simulink model "rlAgentLCLatConstantVxSUMO"  (R2024a)
settings: Solver=VariableStepAuto  StartTime=0.0  StopTime=Tf  FixedStep=1e-3  MaxStep=0.1  RelTol=1e-3
values from neighbouring files (symbols this model uses):
  A = [0 0 0 0 1 -43.6764705882 0 -6.44154540893 0 436.764705882 0 64.4154540893 ... (16 elements, 4x4)]    [DDPGTrain4PingWang.mat]    (also in rlAgentLCParams.m = [)
  Alo = [0  1; 0  0]    [DDPGTrain1.mat]    (also in DDPGTrain2.mat; DDPGTrain4PingWang.mat; rlAgentLCParams.m = [0 1; 0 0])
  B = [0 222.058823529 0 219.719016558]    [DDPGTrain4PingWang.mat]    (also in rlAgentLCParams.m = [0 2*Cf/m 0 2*lf*Cf/Iz]')
  Blo = [0 0.000735294117647]    [DDPGTrain1.mat]    (also in DDPGTrain2.mat; DDPGTrain4PingWang.mat; rlAgentLCParams.m = [0; 1/m])
  Cf = 151000    [DDPGTrain1.mat]    (also in DDPGTrain2.mat; DDPGTrain4PingWang.mat; rlAgentLCParams.m)
  Cr = 146000    [DDPGTrain1.mat]    (also in DDPGTrain2.mat; DDPGTrain4PingWang.mat; rlAgentLCParams.m)
  Iz = 1993    [DDPGTrain1.mat]    (also in DDPGTrain2.mat; DDPGTrain4PingWang.mat; rlAgentLCParams.m)
  Klat = [4.4458 1.2388 123.2048 53.8168]    [DDPGTrain1.mat]    (also in DDPGTrain2.mat; DDPGTrain4PingWang.mat; rlAgentLCParams.m = [4.4458,    1.2388,  123.2048,   53.8168])
  Klo = [4.4721 110.3821]    [DDPGTrain1.mat]    (also in DDPGTrain2.mat; DDPGTrain4PingWang.mat; rlAgentLCParams.m = [4.4721, 110.3821])
  lf = 1.45    [DDPGTrain1.mat]    (also in DDPGTrain2.mat; DDPGTrain4PingWang.mat; rlAgentLCParams.m)
  lr = 1.06    [DDPGTrain1.mat]    (also in DDPGTrain2.mat; DDPGTrain4PingWang.mat; rlAgentLCParams.m)
  m = 1360    [DDPGTrain1.mat]    (also in DDPGTrain2.mat; DDPGTrain4PingWang.mat; rlAgentLCParams.m)
  Ts = 0.11    [DDPGTrain1.mat]    (also in DDPGTrain2.mat; DDPGTrain4PingWang.mat = 0.1; rlAgentLCParams.m = 0.1)
  Vx = 10    [DDPGTrain4PingWang.mat]    (also in rlAgentLCParams.m)
undefined symbols (not defined in the file or in its folder): DiscIntNeverNeededParam
libraries: rllib x1, matrix_library x1
settings Model: Creator=The MathWorks, Inc.  LastModifiedBy=canlab
settings SolverCC: AlgebraicLoopSolver=TrustRegion
settings DataIOCC: SaveOutput=off  SignalLogging=off  DSMLogging=off  SaveTime=off  ReturnWorkspaceOutputs=off
settings DebuggingCC: ParameterPrecisionLossMsg=none  UnconnectedInputMsg=warning  UnconnectedOutputMsg=warning  UnconnectedLineMsg=warning  ArithmeticOperatorsInVariantConditions=warning
settings ModelReferenceCC: EnableRefExpFcnMdlSchedulingChecks=on
settings SFSimCC: SimUseLocalCustomCode=off
settings RTWCC: RTWUseLocalCustomCode=off  GPUComputeCapability=3.5  DLArmComputeVersion=19.05

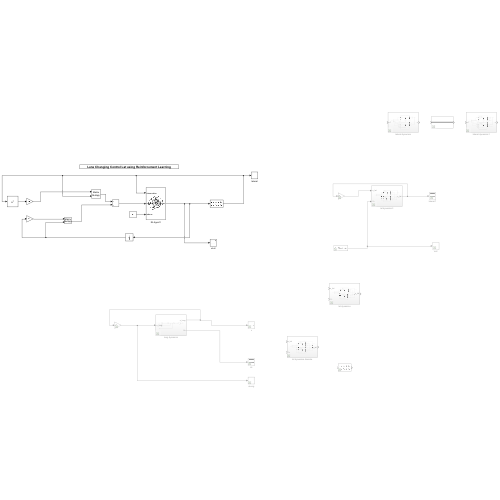
[thumbnail: Simulink's stored preview of the top-level diagram]
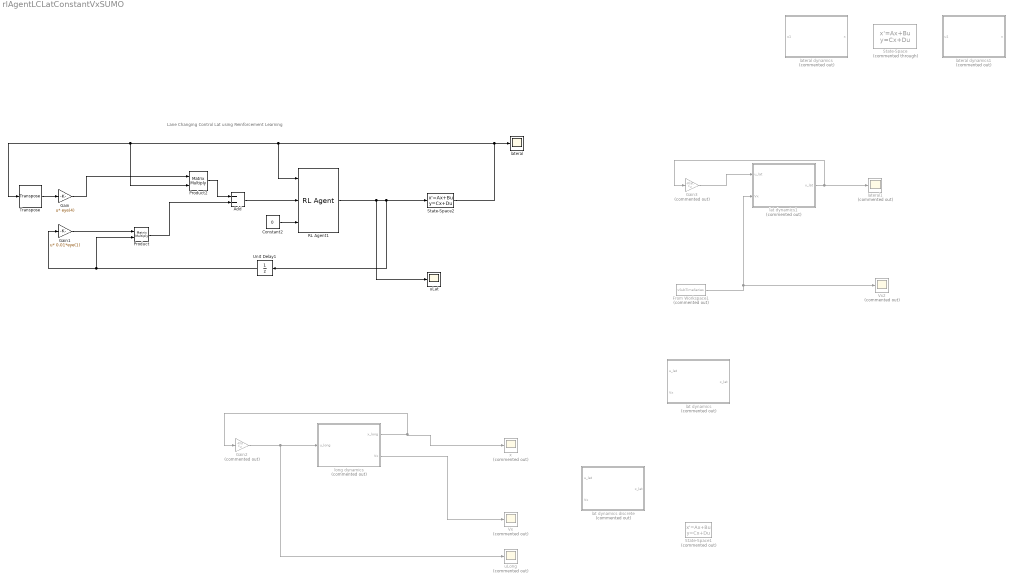
== system rlAgentLCLatConstantVxSUMO ==
  note: Lane Changing Control Lat using Reinforcement Learning
  Add : Sum  Inputs=--
  Constant2 : Constant  Value=0  SampleTime=Ts
  From Workspace1 : FromWorkspace  Commented=on  VariableName=vSubTimeSeries  SampleTime=Ts
  Gain : Gain  Gain=eye(4)  Multiplication=Matrix(u*K)
  Gain1 : Gain  Gain=0.01*eye(1)  Multiplication=Matrix(u*K)
  Gain2 : Gain  Commented=on  Gain=-Klo  Multiplication=Matrix(K*u)
  Gain3 : Gain  Commented=on  Gain=-Klat  Multiplication=Matrix(K*u)
  Product : Product  Multiplication=Matrix(*)
  Product2 : Product  Multiplication=Matrix(*)
  RL Agent1 : rllib/RL Agent  Agent=agent1  ExternalActionAsInput=off  ProvideLastAction=off  ProvideCumRwd=off  TreatAsDirectFeedthrough=on  UseStrictObservationDataTypes=off
  State-Space : StateSpace  Commented=through  A=A  B=B  C=eye(4)  D=zeros(4,1)  InitialCondition=[1;0;1;0]
  State-Space1 : StateSpace  Commented=on  A=Alo  B=Blo  C=eye(2)  D=zeros(2,1)  InitialCondition=[1;20]
  State-Space2 : StateSpace  A=A  B=B  C=eye(4)  D=zeros(4,1)  InitialCondition=[3;0;-0.02;0]
  Transpose : matrix_library/Transpose
  Unit Delay1 : UnitDelay  SampleTime=-1  HasFrameUpgradeWarning=on
  Vx : Scope  Commented=on
  Vx2 : Scope  Commented=on
  lat dynamics : Subsystem  Commented=on
  lat dynamics discrete : Subsystem  Commented=on
  lat dynamics1 : Subsystem  Commented=on
  lateral : Scope
  lateral dynamics : Subsystem  Commented=on
  lateral dynamics1 : Subsystem  Commented=on
  lateral1 : Scope  Commented=on
  long dynamics : Subsystem  Commented=on
  uLat : Scope
  uLong : Scope  Commented=on
  x : Scope  Commented=on
  wires:
  Transpose/1 -> Gain/1
  Product2/1 -> Add/1
  Constant2/1 -> RL Agent1/3
  Add/1 -> RL Agent1/2
  Product/1 -> Add/2
  Unit Delay1/1 -> Product/2, Gain1/1
  Gain/1 -> Product2/1
  Gain1/1 -> Product/1
  Gain2/1 -> long dynamics/1(u_long), uLong/1
  long dynamics/1(x_long) -> x/1, Gain2/1
  long dynamics/2(Vx) -> Vx/1
  RL Agent1/1 -> uLat/1, State-Space2/1, Unit Delay1/1
  From Workspace1/1 -> Vx2/1, lat dynamics1/2(Vx)
  lat dynamics1/1(x_lat) -> lateral1/1, Gain3/1
  Gain3/1 -> lat dynamics1/1(u_lat)
  State-Space2/1 -> Transpose/1, Product2/2, RL Agent1/1, lateral/1

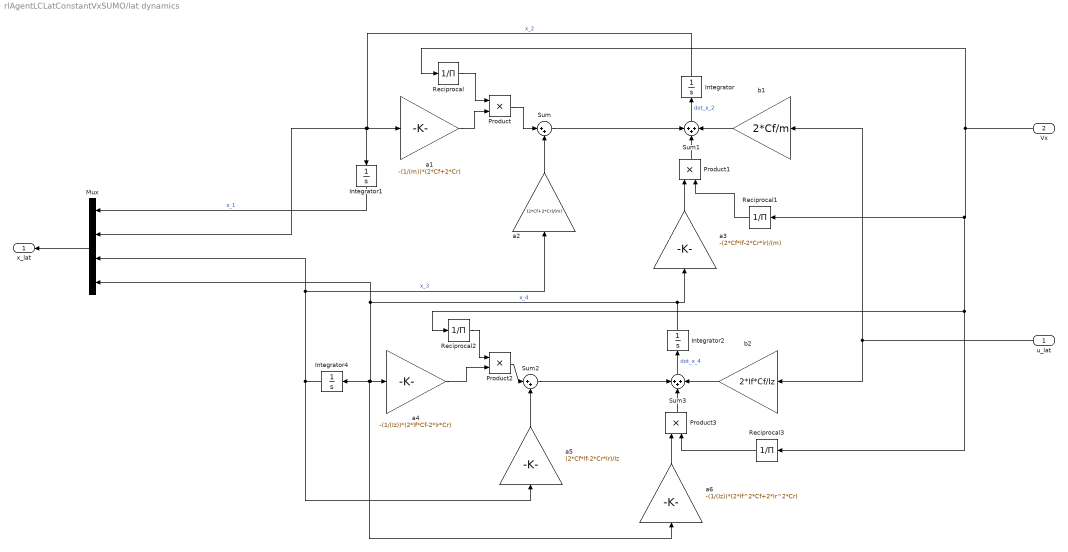
== system rlAgentLCLatConstantVxSUMO/lat dynamics ==
  u_lat : Inport
  Vx : Inport  Port=2
  Integrator : Integrator
  Integrator1 : Integrator  InitialCondition=3.61161063538012
  Integrator2 : Integrator
  Integrator4 : Integrator  InitialCondition=-0.00270532325552732
  Mux : Mux
  Product{,1..3} (4 alike) : Product
  Reciprocal{,1..3} (4 alike) : Product  Inputs=/
  Sum : Sum  Inputs=|++
  Sum1 : Sum  Inputs=+++
  Sum2 : Sum  Inputs=|++
  Sum3 : Sum  Inputs=+++
  a1 : Gain  Gain=-(1/(m))*(2*Cf+2*Cr)
  a2 : Gain  Gain=(2*Cf+2*Cr)/(m)
  a3 : Gain  Gain=-(2*Cf*lf-2*Cr*lr)/(m)
  a4 : Gain  Gain=-(1/(Iz))*(2*lf*Cf-2*lr*Cr)
  a5 : Gain  Gain=(2*Cf*lf-2*Cr*lr)/Iz
  a6 : Gain  Gain=-(1/(Iz))*(2*lf^2*Cf+2*lr^2*Cr)
  b1 : Gain  Gain=2*Cf/m
  b2 : Gain  Gain=2*lf*Cf/Iz
  x_lat : Outport
  wires:
  a3/1 -> Product1/1
  Product1/1 -> Sum1/2
  Sum1/1 -> Integrator/1  "dot_x_2"
  Sum3/1 -> Integrator2/1  "dot_x_4"
  Integrator1/1 -> Mux/1  "x_1"
  u_lat/1 -> b1/1, b2/1
  a2/1 -> Sum/2
  Sum2/1 -> Sum3/1
  Integrator2/1 -> a6/1, Integrator4/1, a4/1, Mux/4, a3/1  "x_4"
  a4/1 -> Product2/2
  Integrator4/1 -> a2/1, Mux/3, a5/1  "x_3"
  Integrator/1 -> Mux/2, Integrator1/1, a1/1  "x_2"
  a5/1 -> Sum2/2
  Product3/1 -> Sum3/2
  Product2/1 -> Sum2/1
  Mux/1 -> x_lat/1
  Reciprocal/1 -> Product/1
  b2/1 -> Sum3/3
  a1/1 -> Product/2
  Vx/1 -> Reciprocal2/1, Reciprocal3/1, Reciprocal1/1, Reciprocal/1
  Reciprocal2/1 -> Product2/1
  Reciprocal1/1 -> Product1/2
  Product/1 -> Sum/1
  Sum/1 -> Sum1/1
  b1/1 -> Sum1/3
  a6/1 -> Product3/1
  Reciprocal3/1 -> Product3/2

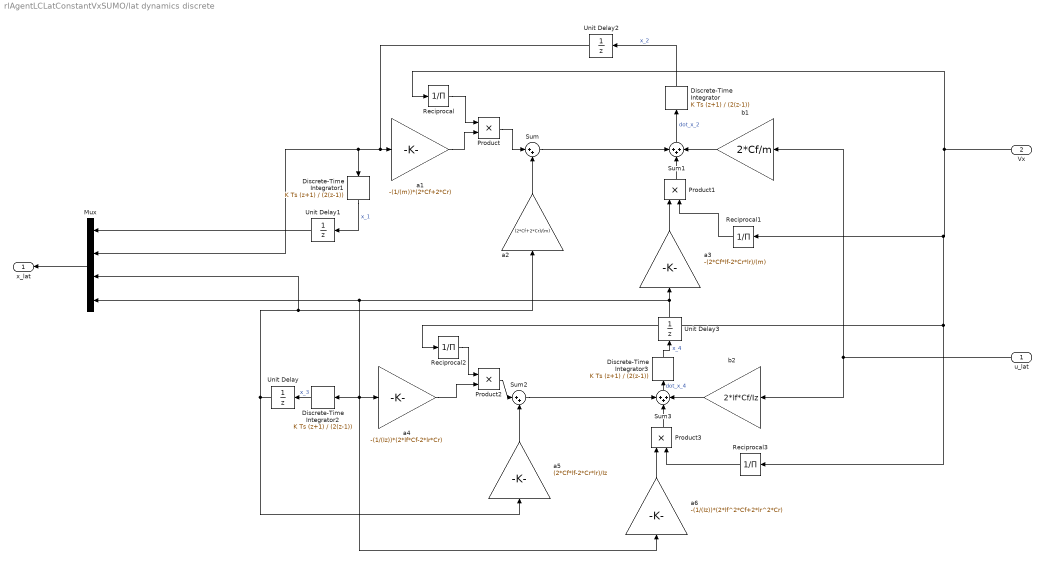
== system rlAgentLCLatConstantVxSUMO/lat dynamics discrete ==
  u_lat : Inport
  Vx : Inport  Port=2
  Discrete-Time Integrator : DiscreteIntegrator  IntegratorMethod=Integration: Trapezoidal  SampleTime=Ts  ICPrevOutput=DiscIntNeverNeededParam  ICPrevScaledInput=DiscIntNeverNeededParam
  Discrete-Time Integrator1 : DiscreteIntegrator  IntegratorMethod=Integration: Trapezoidal  InitialCondition=1  SampleTime=Ts  ICPrevOutput=DiscIntNeverNeededParam  ICPrevScaledInput=DiscIntNeverNeededParam
  Discrete-Time Integrator2 : DiscreteIntegrator  IntegratorMethod=Integration: Trapezoidal  InitialCondition=1  SampleTime=Ts  ICPrevOutput=DiscIntNeverNeededParam  ICPrevScaledInput=DiscIntNeverNeededParam
  Discrete-Time Integrator3 : DiscreteIntegrator  IntegratorMethod=Integration: Trapezoidal  SampleTime=Ts  ICPrevOutput=DiscIntNeverNeededParam  ICPrevScaledInput=DiscIntNeverNeededParam
  Mux : Mux
  Product{,1..3} (4 alike) : Product
  Reciprocal{,1..3} (4 alike) : Product  Inputs=/
  Sum : Sum  Inputs=|++
  Sum1 : Sum  Inputs=+++
  Sum2 : Sum  Inputs=|++
  Sum3 : Sum  Inputs=+++
  Unit Delay{,1..3} (4 alike) : UnitDelay  SampleTime=Ts  HasFrameUpgradeWarning=on
  a1 : Gain  Gain=-(1/(m))*(2*Cf+2*Cr)
  a2 : Gain  Gain=(2*Cf+2*Cr)/(m)
  a3 : Gain  Gain=-(2*Cf*lf-2*Cr*lr)/(m)
  a4 : Gain  Gain=-(1/(Iz))*(2*lf*Cf-2*lr*Cr)
  a5 : Gain  Gain=(2*Cf*lf-2*Cr*lr)/Iz
  a6 : Gain  Gain=-(1/(Iz))*(2*lf^2*Cf+2*lr^2*Cr)
  b1 : Gain  Gain=2*Cf/m
  b2 : Gain  Gain=2*lf*Cf/Iz
  x_lat : Outport
  wires:
  a3/1 -> Product1/1
  Product1/1 -> Sum1/2
  Sum1/1 -> Discrete-Time Integrator/1  "dot_x_2"
  Sum3/1 -> Discrete-Time Integrator3/1  "dot_x_4"
  Discrete-Time Integrator1/1 -> Unit Delay1/1  "x_1"
  u_lat/1 -> b1/1, b2/1
  a2/1 -> Sum/2
  Sum2/1 -> Sum3/1
  Discrete-Time Integrator3/1 -> Unit Delay3/1  "x_4"
  a4/1 -> Product2/2
  Discrete-Time Integrator2/1 -> Unit Delay/1  "x_3"
  Discrete-Time Integrator/1 -> Unit Delay2/1  "x_2"
  a5/1 -> Sum2/2
  Product3/1 -> Sum3/2
  Product2/1 -> Sum2/1
  Mux/1 -> x_lat/1
  Reciprocal/1 -> Product/1
  b2/1 -> Sum3/3
  a1/1 -> Product/2
  Vx/1 -> Reciprocal3/1, Reciprocal2/1, Reciprocal1/1, Reciprocal/1
  Reciprocal2/1 -> Product2/1
  Reciprocal1/1 -> Product1/2
  Product/1 -> Sum/1
  Sum/1 -> Sum1/1
  b1/1 -> Sum1/3
  a6/1 -> Product3/1
  Reciprocal3/1 -> Product3/2
  Unit Delay2/1 -> Discrete-Time Integrator1/1, Mux/2, a1/1
  Unit Delay1/1 -> Mux/1
  Unit Delay/1 -> a5/1, a2/1, Mux/3
  Unit Delay3/1 -> a3/1, a4/1, Discrete-Time Integrator2/1, a6/1, Mux/4

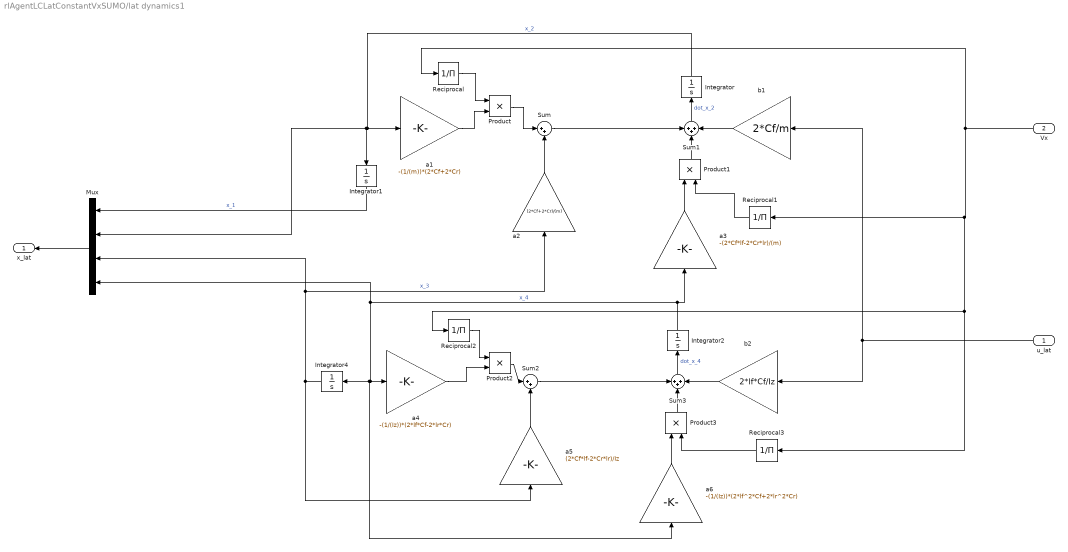
== system rlAgentLCLatConstantVxSUMO/lat dynamics1 ==
  u_lat : Inport
  Vx : Inport  Port=2
  Integrator : Integrator
  Integrator1 : Integrator  InitialCondition=1
  Integrator2 : Integrator
  Integrator4 : Integrator  InitialCondition=1
  Mux : Mux
  Product{,1..3} (4 alike) : Product
  Reciprocal{,1..3} (4 alike) : Product  Inputs=/
  Sum : Sum  Inputs=|++
  Sum1 : Sum  Inputs=+++
  Sum2 : Sum  Inputs=|++
  Sum3 : Sum  Inputs=+++
  a1 : Gain  Gain=-(1/(m))*(2*Cf+2*Cr)
  a2 : Gain  Gain=(2*Cf+2*Cr)/(m)
  a3 : Gain  Gain=-(2*Cf*lf-2*Cr*lr)/(m)
  a4 : Gain  Gain=-(1/(Iz))*(2*lf*Cf-2*lr*Cr)
  a5 : Gain  Gain=(2*Cf*lf-2*Cr*lr)/Iz
  a6 : Gain  Gain=-(1/(Iz))*(2*lf^2*Cf+2*lr^2*Cr)
  b1 : Gain  Gain=2*Cf/m
  b2 : Gain  Gain=2*lf*Cf/Iz
  x_lat : Outport
  wires:
  a3/1 -> Product1/1
  Product1/1 -> Sum1/2
  Sum1/1 -> Integrator/1  "dot_x_2"
  Sum3/1 -> Integrator2/1  "dot_x_4"
  Integrator1/1 -> Mux/1  "x_1"
  u_lat/1 -> b1/1, b2/1
  a2/1 -> Sum/2
  Sum2/1 -> Sum3/1
  Integrator2/1 -> a6/1, Integrator4/1, a4/1, Mux/4, a3/1  "x_4"
  a4/1 -> Product2/2
  Integrator4/1 -> a2/1, Mux/3, a5/1  "x_3"
  Integrator/1 -> Mux/2, Integrator1/1, a1/1  "x_2"
  a5/1 -> Sum2/2
  Product3/1 -> Sum3/2
  Product2/1 -> Sum2/1
  Mux/1 -> x_lat/1
  Reciprocal/1 -> Product/1
  b2/1 -> Sum3/3
  a1/1 -> Product/2
  Vx/1 -> Reciprocal2/1, Reciprocal3/1, Reciprocal1/1, Reciprocal/1
  Reciprocal2/1 -> Product2/1
  Reciprocal1/1 -> Product1/2
  Product/1 -> Sum/1
  Sum/1 -> Sum1/1
  b1/1 -> Sum1/3
  a6/1 -> Product3/1
  Reciprocal3/1 -> Product3/2

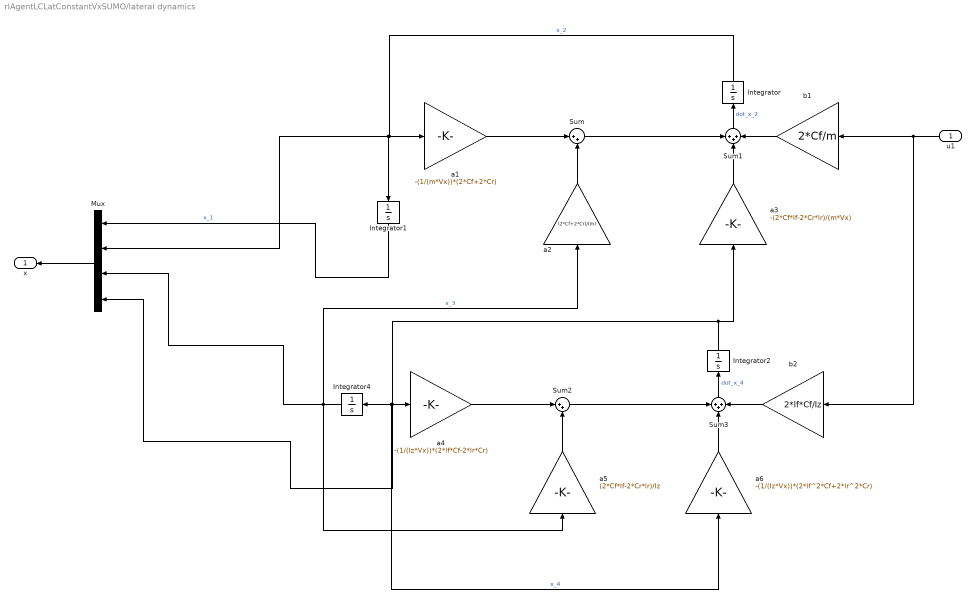
== system rlAgentLCLatConstantVxSUMO/lateral dynamics ==
  u1 : Inport
  Integrator : Integrator
  Integrator1 : Integrator  InitialCondition=1
  Integrator2 : Integrator
  Integrator4 : Integrator  InitialCondition=1
  Mux : Mux
  Sum : Sum  Inputs=|++
  Sum1 : Sum  Inputs=+++
  Sum2 : Sum  Inputs=|++
  Sum3 : Sum  Inputs=+++
  a1 : Gain  Gain=-(1/(m*Vx))*(2*Cf+2*Cr)
  a2 : Gain  Gain=(2*Cf+2*Cr)/(m)
  a3 : Gain  Gain=-(2*Cf*lf-2*Cr*lr)/(m*Vx)
  a4 : Gain  Gain=-(1/(Iz*Vx))*(2*lf*Cf-2*lr*Cr)
  a5 : Gain  Gain=(2*Cf*lf-2*Cr*lr)/Iz
  a6 : Gain  Gain=-(1/(Iz*Vx))*(2*lf^2*Cf+2*lr^2*Cr)
  b1 : Gain  Gain=2*Cf/m
  b2 : Gain  Gain=2*lf*Cf/Iz
  x : Outport
  wires:
  Integrator/1 -> Mux/2, Integrator1/1, a1/1  "x_2"
  a6/1 -> Sum3/2
  Sum/1 -> Sum1/1
  a4/1 -> Sum2/1
  Integrator4/1 -> a5/1, a2/1, Mux/3  "x_3"
  a5/1 -> Sum2/2
  Integrator2/1 -> a6/1, Integrator4/1, a4/1, Mux/4, a3/1  "x_4"
  Sum1/1 -> Integrator/1  "dot_x_2"
  Sum2/1 -> Sum3/1
  Sum3/1 -> Integrator2/1  "dot_x_4"
  b2/1 -> Sum3/3
  b1/1 -> Sum1/3
  a2/1 -> Sum/2
  a3/1 -> Sum1/2
  a1/1 -> Sum/1
  u1/1 -> b2/1, b1/1
  Integrator1/1 -> Mux/1  "x_1"
  Mux/1 -> x/1

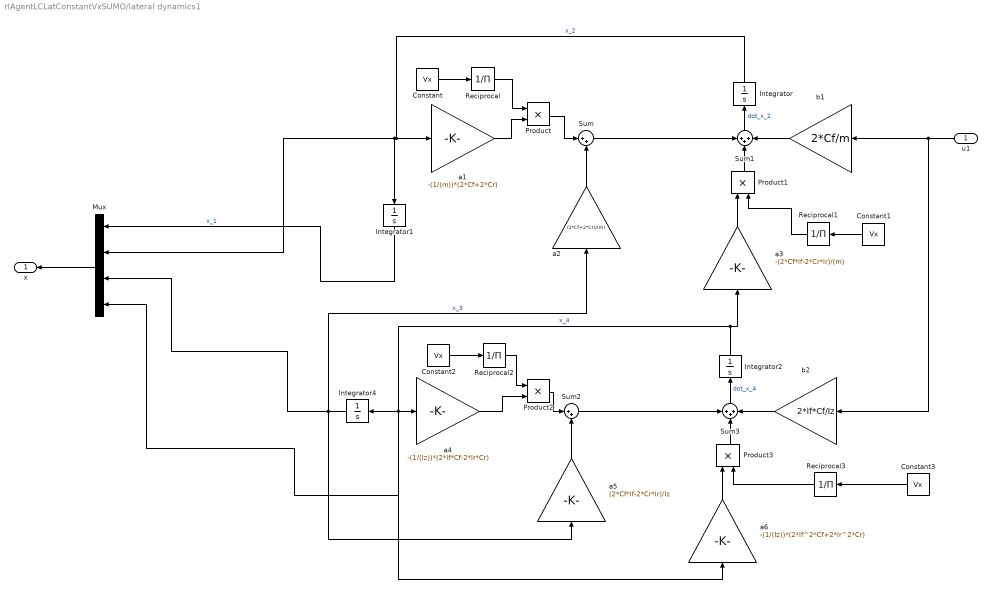
== system rlAgentLCLatConstantVxSUMO/lateral dynamics1 ==
  u1 : Inport
  Constant{,1..3} (4 alike) : Constant  Value=Vx
  Integrator : Integrator
  Integrator1 : Integrator  InitialCondition=1
  Integrator2 : Integrator
  Integrator4 : Integrator  InitialCondition=1
  Mux : Mux
  Product{,1..3} (4 alike) : Product
  Reciprocal{,1..3} (4 alike) : Product  Inputs=/
  Sum : Sum  Inputs=|++
  Sum1 : Sum  Inputs=+++
  Sum2 : Sum  Inputs=|++
  Sum3 : Sum  Inputs=+++
  a1 : Gain  Gain=-(1/(m))*(2*Cf+2*Cr)
  a2 : Gain  Gain=(2*Cf+2*Cr)/(m)
  a3 : Gain  Gain=-(2*Cf*lf-2*Cr*lr)/(m)
  a4 : Gain  Gain=-(1/(Iz))*(2*lf*Cf-2*lr*Cr)
  a5 : Gain  Gain=(2*Cf*lf-2*Cr*lr)/Iz
  a6 : Gain  Gain=-(1/(Iz))*(2*lf^2*Cf+2*lr^2*Cr)
  b1 : Gain  Gain=2*Cf/m
  b2 : Gain  Gain=2*lf*Cf/Iz
  x : Outport
  wires:
  Integrator/1 -> Mux/2, Integrator1/1, a1/1  "x_2"
  a6/1 -> Product3/1
  Sum/1 -> Sum1/1
  a4/1 -> Product2/2
  Integrator4/1 -> a5/1, a2/1, Mux/3  "x_3"
  a5/1 -> Sum2/2
  Integrator2/1 -> a6/1, Integrator4/1, a4/1, Mux/4, a3/1  "x_4"
  Sum1/1 -> Integrator/1  "dot_x_2"
  Sum2/1 -> Sum3/1
  Sum3/1 -> Integrator2/1  "dot_x_4"
  b2/1 -> Sum3/3
  b1/1 -> Sum1/3
  a2/1 -> Sum/2
  a3/1 -> Product1/1
  a1/1 -> Product/2
  u1/1 -> b2/1, b1/1
  Integrator1/1 -> Mux/1  "x_1"
  Mux/1 -> x/1
  Reciprocal/1 -> Product/1
  Constant/1 -> Reciprocal/1
  Product/1 -> Sum/1
  Constant1/1 -> Reciprocal1/1
  Reciprocal1/1 -> Product1/2
  Product1/1 -> Sum1/2
  Constant2/1 -> Reciprocal2/1
  Reciprocal2/1 -> Product2/1
  Product2/1 -> Sum2/1
  Constant3/1 -> Reciprocal3/1
  Reciprocal3/1 -> Product3/2
  Product3/1 -> Sum3/2

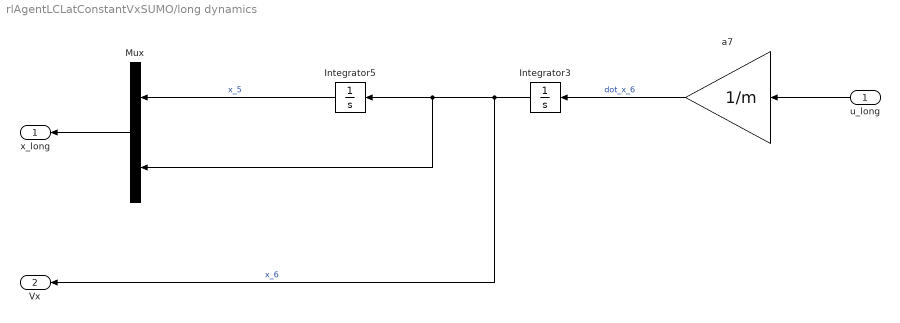
== system rlAgentLCLatConstantVxSUMO/long dynamics ==
  u_long : Inport
  Integrator3 : Integrator  InitialCondition=12
  Integrator5 : Integrator  InitialCondition=1
  Mux : Mux  Inputs=2
  a7 : Gain  Gain=1/m
  x_long : Outport
  Vx : Outport  Port=2
  wires:
  u_long/1 -> a7/1
  a7/1 -> Integrator3/1  "dot_x_6"
  Integrator3/1 -> Vx/1, Mux/2, Integrator5/1  "x_6"
  Integrator5/1 -> Mux/1  "x_5"
  Mux/1 -> x_long/1
